simulink model "TwentyFive"  (R2022b)
settings: Solver=VariableStepAuto  StartTime=0.0  StopTime=10.0  RelTol=1e-3
settings Model: Creator=yeyi5  LastModifiedBy=yeyi5

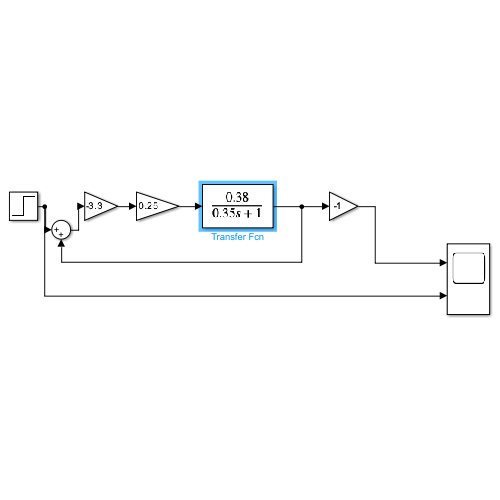
[thumbnail: Simulink's stored preview of the top-level diagram]
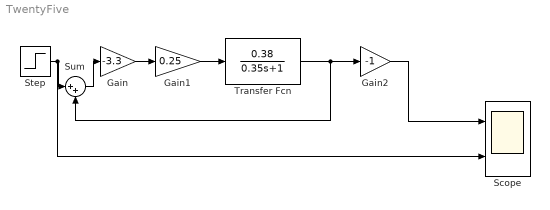
== system TwentyFive ==
  Gain : Gain  Gain=-3.3
  Gain1 : Gain  Gain=0.25
  Gain2 : Gain  Gain=-1
  Scope : Scope  NumInputPorts=2
  Step : Step  After=6  SampleTime=0
  Sum : Sum  Inputs=|++
  Transfer Fcn : TransferFcn  Numerator=[0.38]  Denominator=[0.35 1]
  wires:
  Step/1 -> Scope/2, Sum/1
  Gain/1 -> Gain1/1
  Gain1/1 -> Transfer Fcn/1
  Sum/1 -> Gain/1
  Transfer Fcn/1 -> Sum/2, Gain2/1
  Gain2/1 -> Scope/1
